simulink model "s3eig"  (Simulink 2.00)
settings: Solver=ode15s  StartTime=0.0  StopTime=99  MaxStep=0.0005  RelTol=1e-6  AbsTol=1e-6
values from neighbouring files (symbols this model uses):
  delio = x(3)    [M1.M]    (also in M3.M = delta4; M3G.M = delta4; M4.M = delta)
  Domega = 0    [I3ESSR.M]    (also in M3.M; M3G.M; M5.M = 1; SET1.M = 2)
  H_m = Qbar'*H*Qbar    [M3.M]    (also in M3G.M)
  Id = - Iqo*sin(delio) + Ido*cos(delio)    [M3.M]    (also in M3G.M)
  Iq = Iqo*cos(delio) + Ido*sin(delio)    [M3.M]    (also in M3G.M)
  k = logspace(0,5,1000)    [M1.M]    (also in M4COMP.M = [10:10:300])
  Psido = xls*(-Ido) + Psiado    [M1.M]    (also in M3.M = xls*(-Ido) + Psimdo; M3G.M = xls*(-Ido) + Psimdo; M5.M = Psiado)
  Psifo = xplf*Ifo + Psiado    [M1.M]    (also in M3.M = xplf*Ifo + Psimdo; M3G.M = xplf*Ifo + Psimdo)
  Psikdo = Psiado    [M1.M]    (also in M3.M = Psimdo; M3G.M = Psimdo)
  Psikq2o = Psimqo    [M3.M]    (also in M3G.M)
  Psikqo = Psiaqo    [M1.M]    (also in M3.M = Psimqo; M3G.M = Psimqo)
  Psiqo = xls*(-Iqo) + Psiaqo    [M1.M]    (also in M3.M = xls*(-Iqo) + Psimqo; M3G.M = xls*(-Iqo) + Psimqo; M5.M = 0)
  rpf = rpf/Zbase    [M1.M]    (also in M3.M = 0.00140586866398; M3G.M = 0.00140586866398)
  rpkd = rpkd/Zbase    [M1.M]    (also in M3.M = 0.00408497687269; M3G.M = 0.00408497687269)
  rpkq = rpkq/Zbase    [M1.M]    (also in M3.M = 0.00822300539308; M3G.M = 0.00822300539308)
  rpkq2 = 5.3/wb    (= 0.0140586866398)    [M3.M]    (also in M3G.M)
  rs = 0.00    (= 0)    [I3ESSR.M]    (also in M1.M = rs/Zbase; M3.M; M3G.M = 0.001; M5.M = rs/Zb)
  thetam2to6o = theta_m(2:6)    [M3.M]    (also in M3G.M)
  Vd1 = - Vqo*sin(delio) + Vdo*cos(delio)    [M3.M]    (also in M3G.M)
  VdCs = - Iq*xc(1)    [M3.M]    (also in M3G.M)
  Vq1 = Vqo*cos(delio) + Vdo*sin(delio)    [M3.M]    (also in M3G.M)
  VqCs = Id*xc(1)    [M3.M]    (also in M3G.M)
  wb = wbase    [M1.M]    (also in M2.M = 376.991118431; M3.M = 376.991118431; M3G.M = 376.991118431; M4.M = we)
  wmi_wmi = wmi.*wmi    [M3.M]    (also in M3G.M)
  wmi_xi_2 = wmi_xi_2t'    [M3.M]    (also in M3G.M)
  xls = 0.13    [I3ESSR.M]    (also in M1.M = xls/Zbase; M3.M; M3G.M; M5.M = xls/Zb)
  xmd = xmd/Zbase    [M1.M]    (also in M3.M = 1.66; M3G.M = 1.66; M5.M = xmd/Zb)
  xMD = (1/xls + 1/xmd + 1/xplf + 1/xplkd)^(-1)    [M1.M]    (also in M3.M = 0.00484867453082; M3G.M = 0.00484867453082; M5.M = 0.0152325462012)
  xMQ = (1/xls + 1/xmq + 1/xplkq)^(-1)    [M1.M]    (also in M3.M = 0.0456224786115; M3G.M = 0.0456224786115; M5.M = 0.0170549070248)
  xplf = xplf/Zbase    [M1.M]    (also in M3.M = 0.062; M3G.M = 0.062)
  xplkd = xplkd/Zbase    [M1.M]    (also in M3.M = 0.0055; M3G.M = 0.0055)
  xplkq = xplkq/Zbase    [M1.M]    (also in M3.M = 0.095; M3G.M = 0.095)
  xplkq2 = 0.326    [M3.M]    (also in M3G.M)
undefined symbols (not defined in the file or in its folder): r, xc, xl
settings Model: SaveTime=off  SaveOutput=off  ConsistencyChecking=off

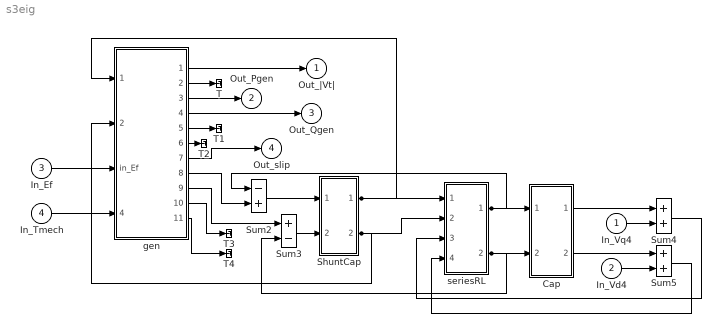
== system s3eig ==
  In_Vq4 : Inport  Port=1  PortWidth=-1  SampleTime=-1
  In_Vd4 : Inport  Port=2  PortWidth=-1  SampleTime=-1
  In_Ef : Inport  Port=3  PortWidth=-1  SampleTime=-1
  In_Tmech : Inport  Port=4  PortWidth=-1  SampleTime=-1
  Cap : Subsystem
  ShuntCap : Subsystem
  Sum2 : Sum  Inputs=-+
  Sum3 : Sum  Inputs=+-
  Sum4 : Sum  Inputs=++
  Sum5 : Sum  Inputs=++
  T{,1..4} (5 alike) : Terminator
  gen : Subsystem
  seriesRL : Subsystem
  Out_|Vt| : Outport  Port=1  InitialOutput=0
  Out_Pgen : Outport  Port=2  InitialOutput=0
  Out_Qgen : Outport  Port=3  InitialOutput=0
  Out_slip : Outport  Port=4  InitialOutput=0
  wires:
  Sum3/1 -> ShuntCap/2(in_ida2b)
  Sum2/1 -> ShuntCap/1(in_iqa2b)
  seriesRL/1(out_iqa2b) -> Cap/1(in_iqa2b), Sum2/1
  seriesRL/2(out_ida2b) -> Cap/2(in_ida2b), Sum3/2
  ShuntCap/1(out_vqa2b) -> seriesRL/1(in_vqa), gen/1(in_vqse)
  ShuntCap/2(out_vda2b) -> seriesRL/2(in_vda), gen/2(in_vdse)
  In_Ef/1 -> gen/3(in_Ef)
  In_Tmech/1 -> gen/4(in_Tmech)
  gen/3(out_Pgen) -> Out_Pgen/1
  gen/4(out_Qgen) -> Out_Qgen/1
  Cap/1(out_vqa2b) -> Sum4/1
  Cap/2(out_vda2b) -> Sum5/1
  Sum4/1 -> seriesRL/3(in_vqb)
  Sum5/1 -> seriesRL/4(in_vdb)
  gen/1(out_|Vt|) -> Out_|Vt|/1
  gen/7(out_(wr-we)/wb) -> Out_slip/1
  gen/8(out_iqe) -> Sum2/2
  gen/9(out_ide) -> Sum3/1
  In_Vq4/1 -> Sum4/2
  In_Vd4/1 -> Sum5/2
  gen/2(out_|It|) -> T/1
  gen/5(out_delta_gen) -> T1/1
  gen/6(out_Tem) -> T2/1
  gen/10(out_LPA-LPB) -> T3/1
  gen/11(out_Gen-Exc) -> T4/1

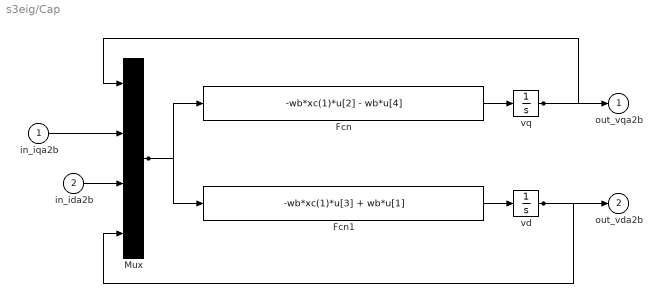
== system s3eig/Cap ==
  in_iqa2b : Inport  Port=1  PortWidth=-1  SampleTime=-1
  in_ida2b : Inport  Port=2  PortWidth=-1  SampleTime=-1
  Fcn : Fcn  Expr=-wb*xc(1)*u[2] - wb*u[4]
  Fcn1 : Fcn  Expr=-wb*xc(1)*u[3] + wb*u[1]
  Mux : Mux  Inputs=4
  vd : Integrator  ExternalReset=none  InitialConditionSource=internal  InitialCondition=VdCs  LimitOutput=off  UpperSaturationLimit=inf  LowerSaturationLimit=-inf  ShowSaturationPort=off  ShowStatePort=off  AbsoluteTolerance=auto
  vq : Integrator  ExternalReset=none  InitialConditionSource=internal  InitialCondition=VqCs  LimitOutput=off  UpperSaturationLimit=inf  LowerSaturationLimit=-inf  ShowSaturationPort=off  ShowStatePort=off  AbsoluteTolerance=auto
  out_vqa2b : Outport  Port=1  InitialOutput=0
  out_vda2b : Outport  Port=2  InitialOutput=0
  wires:
  Fcn1/1 -> vd/1
  Fcn/1 -> vq/1
  Mux/1 -> Fcn1/1, Fcn/1
  vq/1 -> Mux/1, out_vqa2b/1
  in_iqa2b/1 -> Mux/2
  in_ida2b/1 -> Mux/3
  vd/1 -> out_vda2b/1, Mux/4

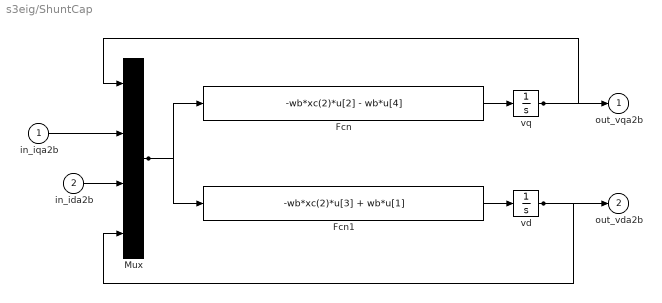
== system s3eig/ShuntCap ==
  in_iqa2b : Inport  Port=1  PortWidth=-1  SampleTime=-1
  in_ida2b : Inport  Port=2  PortWidth=-1  SampleTime=-1
  Fcn : Fcn  Expr=-wb*xc(2)*u[2] - wb*u[4]
  Fcn1 : Fcn  Expr=-wb*xc(2)*u[3] + wb*u[1]
  Mux : Mux  Inputs=4
  vd : Integrator  ExternalReset=none  InitialConditionSource=internal  InitialCondition=Vd1  LimitOutput=off  UpperSaturationLimit=inf  LowerSaturationLimit=-inf  ShowSaturationPort=off  ShowStatePort=off  AbsoluteTolerance=auto
  vq : Integrator  ExternalReset=none  InitialConditionSource=internal  InitialCondition=Vq1  LimitOutput=off  UpperSaturationLimit=inf  LowerSaturationLimit=-inf  ShowSaturationPort=off  ShowStatePort=off  AbsoluteTolerance=auto
  out_vqa2b : Outport  Port=1  InitialOutput=0
  out_vda2b : Outport  Port=2  InitialOutput=0
  wires:
  Fcn1/1 -> vd/1
  Fcn/1 -> vq/1
  Mux/1 -> Fcn1/1, Fcn/1
  vq/1 -> Mux/1, out_vqa2b/1
  in_iqa2b/1 -> Mux/2
  in_ida2b/1 -> Mux/3
  vd/1 -> out_vda2b/1, Mux/4

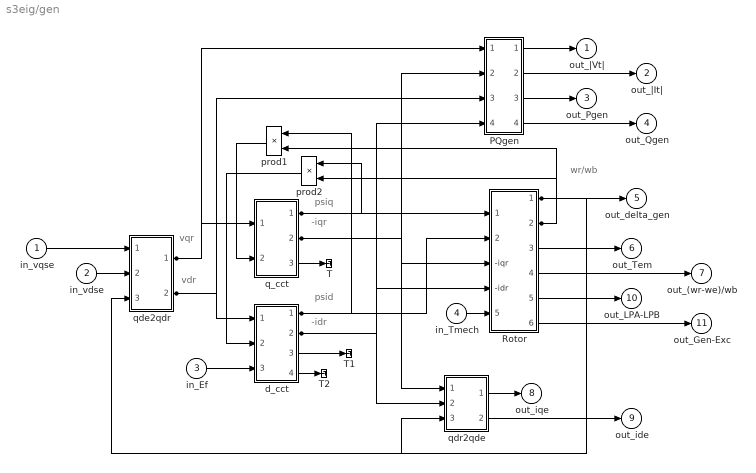
== system s3eig/gen ==
  note: vdr
  note: vqr
  note: wr/wb
  note: psid
  note: psiq
  note: -iqr
  note: -idr
  in_vqse : Inport  Port=1  PortWidth=-1  SampleTime=-1
  in_vdse : Inport  Port=2  PortWidth=-1  SampleTime=-1
  in_Ef : Inport  Port=3  PortWidth=-1  SampleTime=-1
  in_Tmech : Inport  Port=4  PortWidth=-1  SampleTime=-1
  PQgen : Subsystem
  Rotor : Subsystem
  T : Terminator
  T1 : Terminator
  T2 : Terminator
  d_cct : Subsystem
  prod1 : Product  Orientation=left  Inputs=2
  prod2 : Product  Orientation=left  Inputs=2
  q_cct : Subsystem
  qde2qdr : Subsystem
  qdr2qde : Subsystem
  out_|Vt| : Outport  Port=1  InitialOutput=0
  out_|It| : Outport  Port=2  InitialOutput=0
  out_Pgen : Outport  Port=3  InitialOutput=0
  out_Qgen : Outport  Port=4  InitialOutput=0
  out_delta_gen : Outport  Port=5  InitialOutput=0
  out_Tem : Outport  Port=6  InitialOutput=0
  out_(wr-we)/wb : Outport  Port=7  InitialOutput=0
  out_iqe : Outport  Port=8  InitialOutput=0
  out_ide : Outport  Port=9  InitialOutput=0
  out_LPA-LPB : Outport  Port=10  InitialOutput=0
  out_Gen-Exc : Outport  Port=11  InitialOutput=0
  wires:
  Rotor/2("wr/wb ") -> prod1/2, prod2/2
  d_cct/1(Out_psid) -> prod1/1, Rotor/2("psid ")
  prod2/1 -> d_cct/2(In_wrpsiq)
  Rotor/3(Tem) -> out_Tem/1
  in_Ef/1 -> d_cct/3(In_Ef)
  Rotor/4((wr-we)/wb) -> out_(wr-we)/wb/1
  in_Tmech/1 -> Rotor/5(Tmech)
  d_cct/2(Out_-id) -> Rotor/4(-idr), PQgen/4(-idr), qdr2qde/2(-idr)
  qde2qdr/2(vdr) -> d_cct/1(In_vdr), PQgen/3(vdr)
  in_vqse/1 -> qde2qdr/1(vqe)
  in_vdse/1 -> qde2qdr/2(vde)
  Rotor/1(delta_gen) -> out_delta_gen/1, qdr2qde/3(delta), qde2qdr/3("delta ")
  q_cct/2(Out_-iq) -> PQgen/2(-iqr), qdr2qde/1(-iqr), Rotor/3(-iqr)
  q_cct/1(Out_psiq) -> prod2/1, Rotor/1(psiq)
  qdr2qde/1(-iqe) -> out_iqe/1
  qdr2qde/2(-ide) -> out_ide/1
  PQgen/1(Out_|Vt|) -> out_|Vt|/1
  PQgen/3(Pgen) -> out_Pgen/1
  PQgen/4(Qgen) -> out_Qgen/1
  PQgen/2(Out_|It|) -> out_|It|/1
  qde2qdr/1(vqr) -> PQgen/1(vqr), q_cct/1(In_vqr)
  prod1/1 -> q_cct/2(In_wrpsid)
  Rotor/5(LPA-LPB Shaft_torque) -> out_LPA-LPB/1
  Rotor/6(Gen-Exc Shaft_torque) -> out_Gen-Exc/1
  q_cct/3(Out_psimq) -> T/1
  d_cct/3(Out_psimd) -> T1/1
  d_cct/4(Out_ipf) -> T2/1

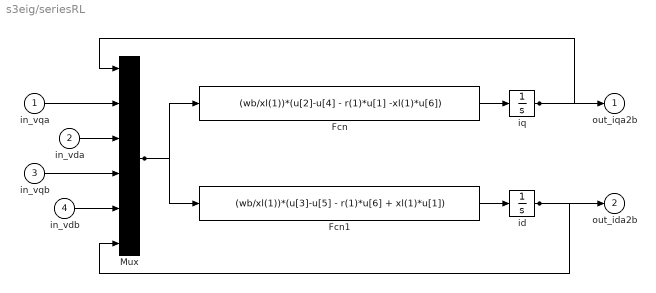
== system s3eig/seriesRL ==
  in_vqa : Inport  Port=1  PortWidth=-1  SampleTime=-1
  in_vda : Inport  Port=2  PortWidth=-1  SampleTime=-1
  in_vqb : Inport  Port=3  PortWidth=-1  SampleTime=-1
  in_vdb : Inport  Port=4  PortWidth=-1  SampleTime=-1
  Fcn : Fcn  Expr=(wb/xl(1))*(u[2]-u[4] - r(1)*u[1] -xl(1)*u[6])
  Fcn1 : Fcn  Expr=(wb/xl(1))*(u[3]-u[5] - r(1)*u[6] + xl(1)*u[1])
  Mux : Mux  Inputs=6
  id : Integrator  ExternalReset=none  InitialConditionSource=internal  InitialCondition=Id  LimitOutput=off  UpperSaturationLimit=inf  LowerSaturationLimit=-inf  ShowSaturationPort=off  ShowStatePort=off  AbsoluteTolerance=auto
  iq : Integrator  ExternalReset=none  InitialConditionSource=internal  InitialCondition=Iq  LimitOutput=off  UpperSaturationLimit=inf  LowerSaturationLimit=-inf  ShowSaturationPort=off  ShowStatePort=off  AbsoluteTolerance=auto
  out_iqa2b : Outport  Port=1  InitialOutput=0
  out_ida2b : Outport  Port=2  InitialOutput=0
  wires:
  Fcn1/1 -> id/1
  Fcn/1 -> iq/1
  Mux/1 -> Fcn1/1, Fcn/1
  iq/1 -> Mux/1, out_iqa2b/1
  in_vqa/1 -> Mux/2
  in_vda/1 -> Mux/3
  in_vqb/1 -> Mux/4
  in_vdb/1 -> Mux/5
  id/1 -> Mux/6, out_ida2b/1

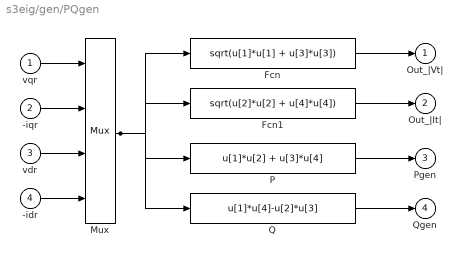
== system s3eig/gen/PQgen ==
  vqr : Inport  Port=1  PortWidth=-1  SampleTime=-1
  -iqr : Inport  Port=2  PortWidth=-1  SampleTime=-1
  vdr : Inport  Port=3  PortWidth=-1  SampleTime=-1
  -idr : Inport  Port=4  PortWidth=-1  SampleTime=-1
  Fcn : Fcn  Expr=sqrt(u[1]*u[1] + u[3]*u[3])
  Fcn1 : Fcn  Expr=sqrt(u[2]*u[2] + u[4]*u[4])
  Mux : Mux  Inputs=4
  P : Fcn  Expr=u[1]*u[2] + u[3]*u[4]
  Q : Fcn  Expr=u[1]*u[4]-u[2]*u[3]
  Out_|Vt| : Outport  Port=1  InitialOutput=0
  Out_|It| : Outport  Port=2  InitialOutput=0
  Pgen : Outport  Port=3  InitialOutput=0
  Qgen : Outport  Port=4  InitialOutput=0
  wires:
  vqr/1 -> Mux/1
  -iqr/1 -> Mux/2
  vdr/1 -> Mux/3
  -idr/1 -> Mux/4
  P/1 -> Pgen/1
  Q/1 -> Qgen/1
  Mux/1 -> P/1, Q/1, Fcn/1, Fcn1/1
  Fcn1/1 -> Out_|It|/1
  Fcn/1 -> Out_|Vt|/1

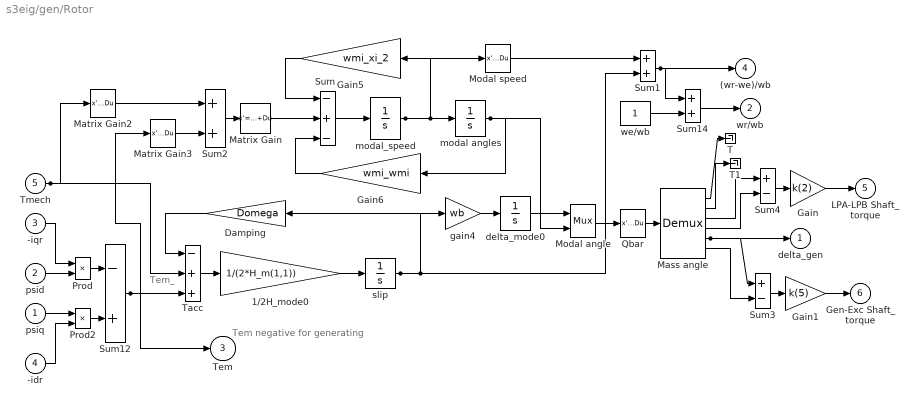
== system s3eig/gen/Rotor ==
  note: Tem_
  note: Tem negative
      |  for generating
  psiq : Inport  Port=1  PortWidth=-1  SampleTime=-1
  "psid " : Inport  Port=2  PortWidth=-1  SampleTime=-1
  -iqr : Inport  Port=3  PortWidth=-1  SampleTime=-1
  -idr : Inport  Port=4  PortWidth=-1  SampleTime=-1
  Tmech : Inport  Port=5  PortWidth=-1  SampleTime=-1
  1/2H_mode0 : Gain  Gain=1/(2*H_m(1,1))
  Damping : Gain  Orientation=left  Gain=Domega
  Gain : Gain  Gain=k(2)
  Gain1 : Gain  Gain=k(5)
  Gain5 : Gain  Orientation=left  Gain=wmi_xi_2
  Gain6 : Gain  Orientation=left  Gain=wmi_wmi
  Mass angle : Demux  Outputs=6
  Matrix Gain : StateSpace  A=[]  B=[]  C=[]  D=K  X0=0  mask(Matrix Gain){@1=tdisk2m}
      mask prompts: @1 "Gain matrix:"
      mask help: Matrix Gain.
      mask init:
      | K = @1;
      mask Help: Multiplies input vector by entered matrix to produce output vector (y=Au).
      mask Display: disp('K')
  Matrix Gain2 : StateSpace  A=[]  B=[]  C=[]  D=K  X0=0  mask(Matrix Gain){@1=tmechv}
      mask prompts: @1 "Gain matrix:"
      mask help: Matrix Gain.
      mask init:
      | K = @1;
      mask Help: Multiplies input vector by entered matrix to produce output vector (y=Au).
      mask Display: disp('K')
  Matrix Gain3 : StateSpace  A=[]  B=[]  C=[]  D=K  X0=0  mask(Matrix Gain){@1=temmask}
      mask prompts: @1 "Gain matrix:"
      mask help: Matrix Gain.
      mask init:
      | K = @1;
      mask Help: Multiplies input vector by entered matrix to produce output vector (y=Au).
      mask Display: disp('K')
  Modal angle : Mux  Inputs=2
  Modal speed : StateSpace  A=[]  B=[]  C=[]  D=K  X0=0  mask(Matrix Gain){@1=omegam2to6}
      mask prompts: @1 "Gain matrix:"
      mask help: Matrix Gain.
      mask init:
      | K = @1;
      mask Help: Multiplies input vector by entered matrix to produce output vector (y=Au).
      mask Display: disp('K')
  Prod : Product  Inputs=2
  Prod2 : Product  Inputs=2
  Qbar : StateSpace  A=[]  B=[]  C=[]  D=K  X0=0  mask(Matrix Gain){@1=Qbar}
      mask prompts: @1 "Gain matrix:"
      mask help: Matrix Gain.
      mask init:
      | K = @1;
      mask Help: Multiplies input vector by entered matrix to produce output vector (y=Au).
      mask Display: disp('K')
  Sum : Sum  Inputs=-+-
  Sum1 : Sum  Inputs=++
  Sum12 : Sum  Inputs=-+
  Sum14 : Sum  Inputs=++
  Sum2 : Sum  Inputs=++
  Sum3 : Sum  Inputs=+-
  Sum4 : Sum  Inputs=+-
  T : Terminator
  T1 : Terminator
  Tacc : Sum  Inputs=-++
  delta_mode0 : Integrator  ExternalReset=none  InitialConditionSource=internal  InitialCondition=delio  LimitOutput=off  UpperSaturationLimit=inf  LowerSaturationLimit=-inf  ShowSaturationPort=off  ShowStatePort=off  AbsoluteTolerance=auto
  gain4 : Gain  Gain=wb
  modal angles : Integrator  ExternalReset=none  InitialConditionSource=internal  InitialCondition=thetam2to6o  LimitOutput=off  UpperSaturationLimit=inf  LowerSaturationLimit=-inf  ShowSaturationPort=off  ShowStatePort=off  AbsoluteTolerance=auto
  modal_speed : Integrator  ExternalReset=none  InitialConditionSource=internal  InitialCondition=[0; 0 ; 0 ;0 ;0 ]  LimitOutput=off  UpperSaturationLimit=inf  LowerSaturationLimit=-inf  ShowSaturationPort=off  ShowStatePort=off  AbsoluteTolerance=auto
  slip : Integrator  ExternalReset=none  InitialConditionSource=internal  InitialCondition=0  LimitOutput=off  UpperSaturationLimit=inf  LowerSaturationLimit=-inf  ShowSaturationPort=off  ShowStatePort=off  AbsoluteTolerance=auto
  we/wb : Constant  Value=1
  delta_gen : Outport  Port=1  InitialOutput=0
  "wr/wb " : Outport  Port=2  InitialOutput=0
  Tem : Outport  Port=3  InitialOutput=0
  (wr-we)/wb : Outport  Port=4  InitialOutput=0
  LPA-LPB Shaft_torque : Outport  Port=5  InitialOutput=0
  Gen-Exc Shaft_torque : Outport  Port=6  InitialOutput=0
  wires:
  Damping/1 -> Tacc/1
  gain4/1 -> delta_mode0/1
  Prod2/1 -> Sum12/2
  1/2H_mode0/1 -> slip/1
  we/wb/1 -> Sum14/2
  Tacc/1 -> 1/2H_mode0/1
  Prod/1 -> Sum12/1
  -iqr/1 -> Prod/1
  "psid "/1 -> Prod/2
  psiq/1 -> Prod2/1
  -idr/1 -> Prod2/2
  Sum14/1 -> "wr/wb "/1
  Sum12/1 -> Tacc/3, Tem/1, Matrix Gain3/1
  Gain5/1 -> Sum/1
  Matrix Gain/1 -> Sum/2
  Sum2/1 -> Matrix Gain/1
  Matrix Gain3/1 -> Sum2/2
  Matrix Gain2/1 -> Sum2/1
  Tmech/1 -> Tacc/2, Matrix Gain2/1
  Sum/1 -> modal_speed/1
  Gain6/1 -> Sum/3
  modal_speed/1 -> Gain5/1, modal angles/1, Modal speed/1
  Sum1/1 -> Sum14/1, (wr-we)/wb/1
  slip/1 -> Damping/1, gain4/1, Sum1/2
  Modal speed/1 -> Sum1/1
  modal angles/1 -> Gain6/1, Modal angle/2
  delta_mode0/1 -> Modal angle/1
  Modal angle/1 -> Qbar/1
  Qbar/1 -> Mass angle/1
  Mass angle/3 -> Sum4/1
  Mass angle/4 -> Sum4/2
  Mass angle/5 -> delta_gen/1, Sum3/1
  Mass angle/6 -> Sum3/2
  Sum4/1 -> Gain/1
  Sum3/1 -> Gain1/1
  Gain/1 -> LPA-LPB Shaft_torque/1
  Gain1/1 -> Gen-Exc Shaft_torque/1
  Mass angle/1 -> T/1
  Mass angle/2 -> T1/1

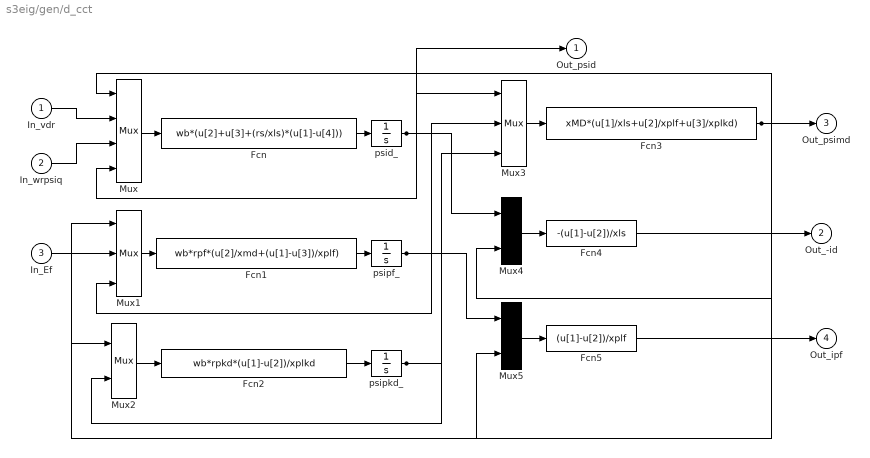
== system s3eig/gen/d_cct ==
  In_vdr : Inport  Port=1  PortWidth=-1  SampleTime=-1
  In_wrpsiq : Inport  Port=2  PortWidth=-1  SampleTime=-1
  In_Ef : Inport  Port=3  PortWidth=-1  SampleTime=-1
  Fcn : Fcn  Expr=wb*(u[2]+u[3]+(rs/xls)*(u[1]-u[4]))
  Fcn1 : Fcn  Expr=wb*rpf*(u[2]/xmd+(u[1]-u[3])/xplf)
  Fcn2 : Fcn  Expr=wb*rpkd*(u[1]-u[2])/xplkd
  Fcn3 : Fcn  Expr=xMD*(u[1]/xls+u[2]/xplf+u[3]/xplkd)
  Fcn4 : Fcn  Expr=-(u[1]-u[2])/xls
  Fcn5 : Fcn  Expr=(u[1]-u[2])/xplf
  Mux : Mux  Inputs=4
  Mux1 : Mux  Inputs=3
  Mux2 : Mux  Inputs=2
  Mux3 : Mux  Inputs=3
  Mux4 : Mux  Inputs=2
  Mux5 : Mux  Inputs=2
  psid_ : Integrator  ExternalReset=none  InitialConditionSource=internal  InitialCondition=Psido  LimitOutput=off  UpperSaturationLimit=inf  LowerSaturationLimit=-inf  ShowSaturationPort=off  ShowStatePort=off  AbsoluteTolerance=auto
  psipf_ : Integrator  ExternalReset=none  InitialConditionSource=internal  InitialCondition=Psifo  LimitOutput=off  UpperSaturationLimit=inf  LowerSaturationLimit=-inf  ShowSaturationPort=off  ShowStatePort=off  AbsoluteTolerance=auto
  psipkd_ : Integrator  ExternalReset=none  InitialConditionSource=internal  InitialCondition=Psikdo  LimitOutput=off  UpperSaturationLimit=inf  LowerSaturationLimit=-inf  ShowSaturationPort=off  ShowStatePort=off  AbsoluteTolerance=auto
  Out_psid : Outport  Port=1  InitialOutput=0
  Out_-id : Outport  Port=2  InitialOutput=0
  Out_psimd : Outport  Port=3  InitialOutput=0
  Out_ipf : Outport  Port=4  InitialOutput=0
  wires:
  In_wrpsiq/1 -> Mux/3
  In_vdr/1 -> Mux/2
  Mux/1 -> Fcn/1
  Fcn/1 -> psid_/1
  Mux1/1 -> Fcn1/1
  Fcn1/1 -> psipf_/1
  In_Ef/1 -> Mux1/2
  Mux2/1 -> Fcn2/1
  Fcn2/1 -> psipkd_/1
  psid_/1 -> Mux/4, Mux3/1, Mux4/1, Out_psid/1
  psipf_/1 -> Mux1/3, Mux3/2, Mux5/1
  psipkd_/1 -> Mux2/2, Mux3/3
  Mux3/1 -> Fcn3/1
  Mux4/1 -> Fcn4/1
  Mux5/1 -> Fcn5/1
  Fcn3/1 -> Mux5/2, Mux4/2, Mux2/1, Mux1/1, Mux/1, Out_psimd/1
  Fcn4/1 -> Out_-id/1
  Fcn5/1 -> Out_ipf/1

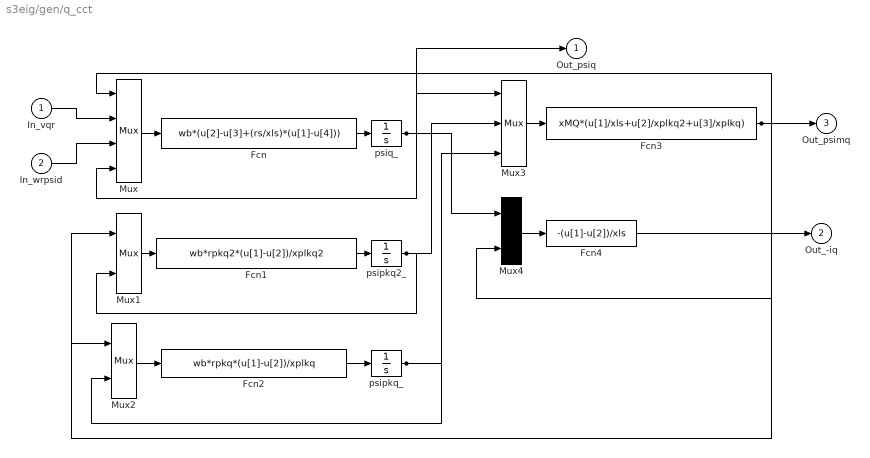
== system s3eig/gen/q_cct ==
  In_vqr : Inport  Port=1  PortWidth=-1  SampleTime=-1
  In_wrpsid : Inport  Port=2  PortWidth=-1  SampleTime=-1
  Fcn : Fcn  Expr=wb*(u[2]-u[3]+(rs/xls)*(u[1]-u[4]))
  Fcn1 : Fcn  Expr=wb*rpkq2*(u[1]-u[2])/xplkq2
  Fcn2 : Fcn  Expr=wb*rpkq*(u[1]-u[2])/xplkq
  Fcn3 : Fcn  Expr=xMQ*(u[1]/xls+u[2]/xplkq2+u[3]/xplkq)
  Fcn4 : Fcn  Expr=-(u[1]-u[2])/xls
  Mux : Mux  Inputs=4
  Mux1 : Mux  Inputs=2
  Mux2 : Mux  Inputs=2
  Mux3 : Mux  Inputs=3
  Mux4 : Mux  Inputs=2
  psipkq2_ : Integrator  ExternalReset=none  InitialConditionSource=internal  InitialCondition=Psikq2o  LimitOutput=off  UpperSaturationLimit=inf  LowerSaturationLimit=-inf  ShowSaturationPort=off  ShowStatePort=off  AbsoluteTolerance=auto
  psipkq_ : Integrator  ExternalReset=none  InitialConditionSource=internal  InitialCondition=Psikqo  LimitOutput=off  UpperSaturationLimit=inf  LowerSaturationLimit=-inf  ShowSaturationPort=off  ShowStatePort=off  AbsoluteTolerance=auto
  psiq_ : Integrator  ExternalReset=none  InitialConditionSource=internal  InitialCondition=Psiqo  LimitOutput=off  UpperSaturationLimit=inf  LowerSaturationLimit=-inf  ShowSaturationPort=off  ShowStatePort=off  AbsoluteTolerance=auto
  Out_psiq : Outport  Port=1  InitialOutput=0
  Out_-iq : Outport  Port=2  InitialOutput=0
  Out_psimq : Outport  Port=3  InitialOutput=0
  wires:
  In_wrpsid/1 -> Mux/3
  In_vqr/1 -> Mux/2
  Mux/1 -> Fcn/1
  Fcn/1 -> psiq_/1
  Mux1/1 -> Fcn1/1
  Fcn1/1 -> psipkq2_/1
  Mux2/1 -> Fcn2/1
  Fcn2/1 -> psipkq_/1
  psiq_/1 -> Mux/4, Mux3/1, Mux4/1, Out_psiq/1
  psipkq_/1 -> Mux2/2, Mux3/3
  Mux3/1 -> Fcn3/1
  Mux4/1 -> Fcn4/1
  Fcn3/1 -> Mux4/2, Mux2/1, Mux1/1, Mux/1, Out_psimq/1
  Fcn4/1 -> Out_-iq/1
  psipkq2_/1 -> Mux3/2, Mux1/2

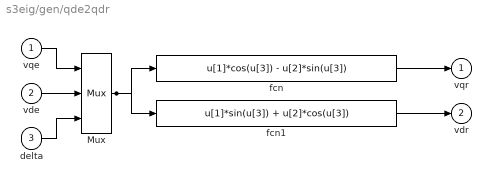
== system s3eig/gen/qde2qdr ==
  vqe : Inport  Port=1  PortWidth=-1  SampleTime=-1
  vde : Inport  Port=2  PortWidth=-1  SampleTime=-1
  "delta " : Inport  Port=3  PortWidth=-1  SampleTime=-1
  Mux : Mux  Inputs=3
  fcn : Fcn  Expr=u[1]*cos(u[3]) - u[2]*sin(u[3])
  fcn1 : Fcn  Expr=u[1]*sin(u[3]) + u[2]*cos(u[3])
  vqr : Outport  Port=1  InitialOutput=0
  vdr : Outport  Port=2  InitialOutput=0
  wires:
  fcn1/1 -> vdr/1
  vqe/1 -> Mux/1
  fcn/1 -> vqr/1
  Mux/1 -> fcn/1, fcn1/1
  "delta "/1 -> Mux/3
  vde/1 -> Mux/2

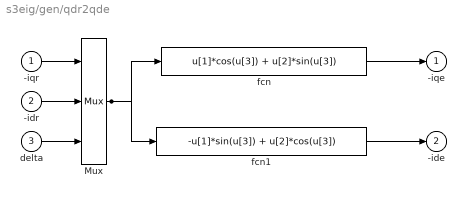
== system s3eig/gen/qdr2qde ==
  -iqr : Inport  Port=1  PortWidth=-1  SampleTime=-1
  -idr : Inport  Port=2  PortWidth=-1  SampleTime=-1
  delta : Inport  Port=3  PortWidth=-1  SampleTime=-1
  Mux : Mux  Inputs=3
  fcn : Fcn  Expr=u[1]*cos(u[3]) + u[2]*sin(u[3])
  fcn1 : Fcn  Expr=-u[1]*sin(u[3]) + u[2]*cos(u[3])
  -iqe : Outport  Port=1  InitialOutput=0
  -ide : Outport  Port=2  InitialOutput=0
  wires:
  fcn1/1 -> -ide/1
  -iqr/1 -> Mux/1
  fcn/1 -> -iqe/1
  Mux/1 -> fcn/1, fcn1/1
  -idr/1 -> Mux/2
  delta/1 -> Mux/3
